simulink model "speed_ctrl_1"  (R2019b)
settings: Solver=ode45  StartTime=0.0  StopTime=1.0  MaxStep=0.001  RelTol=1e-3  EnableMultiTasking=on
undefined symbols (not defined in the file): dist, mot, rads2rpm, rpm2rads, wctrl, wfilt, wref
settings Model: ExtModeAutoUpdateStatusClock=off  Creator=Riccardo  LastModifiedBy=riccardo
settings DataIOCC: LimitDataPoints=on  SaveFormat=Array  SignalLoggingSaveFormat=ModelDataLogs  ReturnWorkspaceOutputs=off
settings OptimizationCC: ExpressionDepthLimit=2147483647  InitFltsAndDblsToZero=on  LifeSpan=inf
settings DebuggingCC: SaveWithParameterizedLinksMsg=none  UnderspecifiedInitializationDetection=Classic  MergeDetectMultiDrivingBlocksExec=none  FcnCallInpInsideContextMsg=warning  StateNameClashWarn=warning  SFUnexpectedBacktrackingDiag=warning  SFNoUnconditionalDefaultTransitionDiag=warning  ArithmeticOperatorsInVariantConditions=warning
settings HardwareCC: ProdBitPerPointer=32  ProdBitPerSizeT=32  ProdBitPerPtrDiffT=32  ProdLargestAtomicFloat=None  ProdIntDivRoundTo=Undefined  ProdEndianess=Unspecified  ProdWordSize=32  ProdHWDeviceType=32-bit Generic
settings ModelReferenceCC: PropagateSignalLabelsOutOfModel=off
settings SFSimCC: SimUseLocalCustomCode=off  CustomCodeUndefinedFunction=UseInterfaceOnly
settings RTWCC: RTWUseLocalCustomCode=off
settings CodeAppCC: StateflowObjectComments=on
settings GRTTargetCC: TargetFcnLib=ansi_tfl_tmw.mat  TargetLangStandard=C89/C90 (ANSI)  GeneratePreprocessorConditionals=Disable all  CombineOutputUpdateFcns=off  GRTInterface=on
settings ConfigComp: CovMetricSettings=dw  CovHtmlReporting=on  CovSaveCumulativeToWorkspaceVar=on  CovSaveSingleToWorkspaceVar=on  CovExternalEMLEnable=off  CovSFcnEnable=off

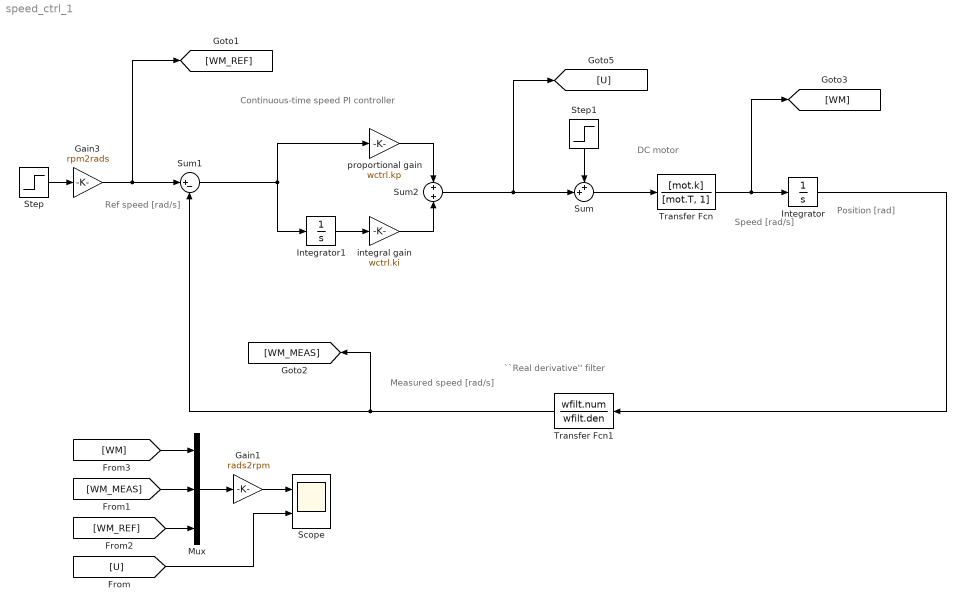
== system speed_ctrl_1 ==
  note: Continuous-time speed PI controller
  note: DC motor
  note: ``Real derivative'' filter
  note: Speed
      | [rad/s]
  note: Measured speed
      | [rad/s]
  note: Position
      | [rad]
  note: Ref speed
      | [rad/s]
  Gain1 : Gain  Gain=rads2rpm
  Gain3 : Gain  Gain=rpm2rads
  Integrator : Integrator
  Integrator1 : Integrator
  Mux : Mux  Inputs=3
  Scope : Scope  NumInputPorts=2
  Step : Step  Time=wref.t0  After=wref.A  SampleTime=0
  Step1 : Step  Time=dist.t0  After=dist.A  SampleTime=0
  Sum : Sum  Inputs=++|
  Sum1 : Sum  Inputs=|+-
  Sum2 : Sum
  Transfer Fcn : TransferFcn  Numerator=[mot.k]  Denominator=[mot.T, 1]
  Transfer Fcn1 : TransferFcn  Numerator=wfilt.num  Denominator=wfilt.den
  integral gain : Gain  Gain=wctrl.ki
  proportional gain : Gain  Gain=wctrl.kp
  wires:
  Transfer Fcn/1 -> [WM], Integrator/1
  Sum/1 -> Transfer Fcn/1
  Integrator1/1 -> integral gain/1
  proportional gain/1 -> Sum2/1
  Sum1/1 -> Integrator1/1, proportional gain/1
  Step/1 -> Gain3/1
  Sum2/1 -> Sum/2, [U]
  Transfer Fcn1/1 -> [WM_MEAS], Sum1/2
  Mux/1 -> Gain1/1
  [U] -> Scope/2
  Integrator/1 -> Transfer Fcn1/1
  Step1/1 -> Sum/1
  [WM_REF] -> Mux/3
  [WM_MEAS] -> Mux/2
  [WM] -> Mux/1
  Gain3/1 -> Sum1/1, [WM_REF]
  integral gain/1 -> Sum2/2
  Gain1/1 -> Scope/1
